simulink model "test_hyst_drift_parallel"  (R2016b)
settings: Solver=VariableStepAuto  StartTime=0.0  StopTime=trun  RelTol=1e-3
values from neighbouring files (symbols this model uses):
  d = self.d    [TestHystDriftParallel.m]    (also in TestPIHyst.m = [dmin, 0, dplus]')
  dp = fi(dp, 1, 16, 11)    [TestHystDriftParallel.m]
  r = self.r    [TestHystDriftParallel.m]    (also in TestPIHyst.m = ([0:nw-1]'./(nw) )*umax)
  rp = fi(rp, 1, 16, 11)    [TestHystDriftParallel.m]
  w = self.w    [TestHystDriftParallel.m]    (also in TestPIHyst.m = [0.0001; 0.02; .4; 0.78; 1; 0.03; 0.04])
  wp = fi(wp, 1, 16, 11)    [TestHystDriftParallel.m]
  ws = self.ws    [TestHystDriftParallel.m]    (also in TestPIHyst.m = [0.0001; 0.02; .3; .5; 1.5; 0.03; .5; .065; 0.04])
  wsp = fi(wsp, 1, 16, 11)    [TestHystDriftParallel.m]
undefined symbols (not defined in the file or in its folder): den, num
libraries: cstblocks x4
settings Model: Creator=arnold  LastModifiedBy=arnold

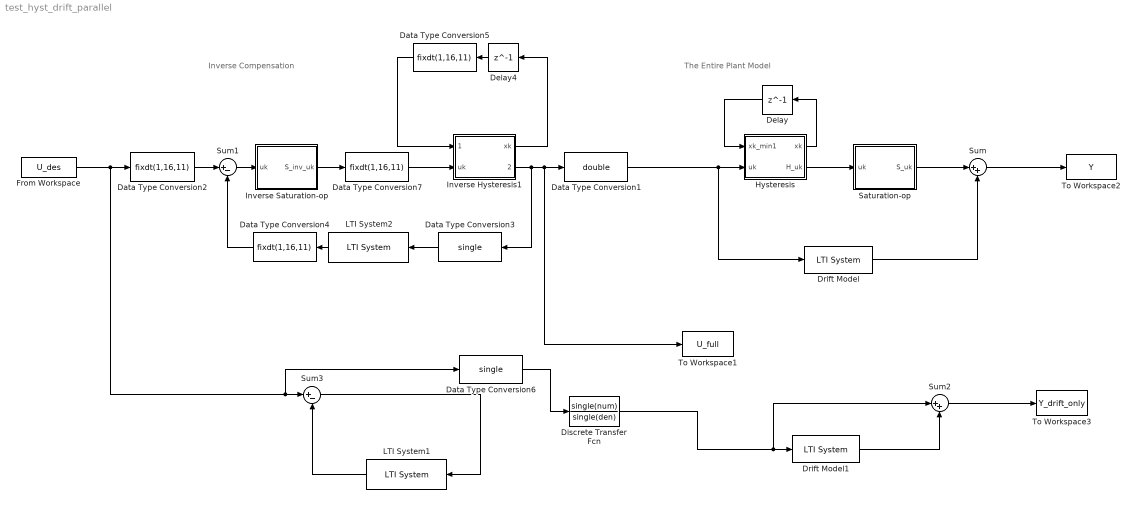
== system test_hyst_drift_parallel ==
  note: The Entire Plant Model
  note: Inverse Compensation
  Data Type Conversion1 : DataTypeConversion  OutDataTypeStr=double  LockScale=on
  Data Type Conversion{2,4..5,7} (4 alike) : DataTypeConversion  OutDataTypeStr=fixdt(1,16,11)
  Data Type Conversion3 : DataTypeConversion  OutDataTypeStr=single  LockScale=on
  Data Type Conversion6 : DataTypeConversion  OutDataTypeStr=single  LockScale=on
  Delay : Delay  DelayLength=1  InitialCondition=zeros(length(r),1)
  Delay4 : Delay  DelayLength=1  InitialCondition=fi(zeros(length(rp),1), 1, 16, 11)
  Discrete Transfer Fcn : DiscreteTransferFcn  Numerator=single(num)  Denominator=single(den)
  Drift Model : cstblocks/LTI System  sys=gdrift  IC=[]
  Drift Model1 : cstblocks/LTI System  sys=gdrift  IC=[]
  From Workspace : FromWorkspace  VariableName=U_des  SampleTime=0
  Hysteresis : MATLAB Function  TreatAsAtomicUnit=on
  Inverse Hysteresis1 : MATLAB Function  TreatAsAtomicUnit=on
  Inverse Saturation-op : MATLAB Function  TreatAsAtomicUnit=on
  LTI System1 : cstblocks/LTI System  sys=gdrift  IC=[]
  LTI System2 : cstblocks/LTI System  sys=gdrift  IC=[]
  Saturation-op : MATLAB Function  TreatAsAtomicUnit=on
  Sum : Sum  Inputs=|++
  Sum1 : Sum  Inputs=|+-  OutDataTypeStr=fixdt(1,16,11)
  Sum2 : Sum  Inputs=|++
  Sum3 : Sum  Inputs=|+-
  To Workspace1 : ToWorkspace  VariableName=U_full  SaveFormat=Timeseries  SampleTime=-1
      settings: Save2DSignal=2-D array (concatenate along first dimension)
  To Workspace2 : ToWorkspace  VariableName=Y  SaveFormat=Timeseries  SampleTime=-1
      settings: Save2DSignal=2-D array (concatenate along first dimension)
  To Workspace3 : ToWorkspace  VariableName=Y_drift_only  SaveFormat=Timeseries  SampleTime=-1
      settings: Save2DSignal=2-D array (concatenate along first dimension)
  wires:
  Drift Model/1 -> Sum/2
  Hysteresis/1(xk) -> Delay/1
  Delay/1 -> Hysteresis/1(xk_min1)
  Hysteresis/2(H_uk) -> Saturation-op/1(uk)
  LTI System2/1 -> Data Type Conversion4/1
  From Workspace/1 -> Data Type Conversion2/1, Data Type Conversion6/1, Sum3/1
  Saturation-op/1(S_uk) -> Sum/1
  Drift Model1/1 -> Sum2/2
  Sum3/1 -> LTI System1/1
  LTI System1/1 -> Sum3/2
  Sum/1 -> To Workspace2/1
  Sum2/1 -> To Workspace3/1
  Inverse Hysteresis1/1(xk) -> Delay4/1
  Data Type Conversion5/1 -> Inverse Hysteresis1/1(xk_min1)
  Inverse Hysteresis1/2(H_inv_uk) -> Data Type Conversion3/1, To Workspace1/1, Data Type Conversion1/1
  Delay4/1 -> Data Type Conversion5/1
  Inverse Saturation-op/1(S_inv_uk) -> Data Type Conversion7/1
  Sum1/1 -> Inverse Saturation-op/1(uk)
  Data Type Conversion3/1 -> LTI System2/1
  Data Type Conversion1/1 -> Drift Model/1, Hysteresis/2(uk)
  Data Type Conversion2/1 -> Sum1/1
  Data Type Conversion4/1 -> Sum1/2
  Discrete Transfer Fcn/1 -> Sum2/1, Drift Model1/1
  Data Type Conversion6/1 -> Discrete Transfer Fcn/1
  Data Type Conversion7/1 -> Inverse Hysteresis1/2(uk)

== matlab function test_hyst_drift_parallel/Inverse Saturation-op ==
  data: uk input; S_inv_uk output fixdt(1,16,11); wsp parameter; dp parameter fixdt(1,16,11)
function S_inv_uk  = fcn(uk, wsp, dp)
  % Implement simple Saturation model.
%   keyboard

  if length(dp) > 1
    Sd_vec = 0*dp(:);
    for i=1:length(dp)
      if dp(i) == 0
        Sd_vec(i) = uk;
      elseif dp(i) > 0
        Sd_vec(i) = max(uk - dp(i), 0);
      else
        Sd_vec(i) = min(uk - dp(i), 0);
      end
    end
    S_inv_uk = wsp(:)'*Sd_vec;
  else
   S_inv_uk = uk;
  end
  S_inv_uk = fi(S_inv_uk, 1, 16, 11);
end

== matlab function test_hyst_drift_parallel/Hysteresis ==
  data: xk output; xk_min1 input; uk input; H_uk output; r parameter; w parameter
function [xk, H_uk] = fcn(xk_min1, uk, r, w)
  % Implement simple IP hysteresis model.
  if length(r) > 1
    xk = r(:)*0;
    for j = 1:length(r)
      xk(j) = max(uk - r(j), min(uk+r(j), xk_min1(j)));
    end
    
    H_uk = w'*xk(:);
  else
    xk = xk_min1;
    H_uk = uk;
  end
end

== matlab function test_hyst_drift_parallel/Inverse Hysteresis1 ==
  data: xk output; xk_min1 input fixdt(1,16,11); uk input; H_inv_uk output; rp parameter; wp parameter
function [xk, H_inv_uk] = fcn(xk_min1, uk, rp, wp)
  % Implement simple IP hysteresis model.
%   keyboard
  if length(rp) > 1
    xk = rp(:)*fi(0, 1, 16, 11);
    for j = 1:length(rp)
      xk(j) = max(uk - rp(j), min(uk+rp(j), xk_min1(j)));
    end
    
    H_inv_uk = wp'*xk(:);
  else
    xk = xk_min1;
    H_inv_uk = uk;
  end
end

== matlab function test_hyst_drift_parallel/Saturation-op ==
  data: uk input; S_uk output; ws parameter; d parameter
function S_uk  = fcn(uk, ws, d)
  % Implement simple Saturation model.
%   keyboard
  if length(d) > 1
    Sd_vec = 0*d(:);
    for i=1:length(d)
      if d(i) == 0
        Sd_vec(i) = uk;
      elseif d(i) > 0
        Sd_vec(i) = max(uk - d(i), 0);
      else
        Sd_vec(i) = min(uk - d(i), 0);
      end
    end
    S_uk = ws(:)'*Sd_vec;
  else
   S_uk = uk;
  end
end
